simulink library "INP_IMU_ManOver"  (R2022a)
settings: Solver=VariableStepAuto  StartTime=0.0  StopTime=10.0  RelTol=1e-3
undefined symbols (not defined in the file): INP_IMU_p_ALatVehLoLim_mps2, INP_IMU_p_ALatVehMan_mps2, INP_IMU_p_ALatVehUpLim_mps2, INP_IMU_p_ALgtVehLoLim_mps2, INP_IMU_p_ALgtVehMan_mps2, INP_IMU_p_ALgtVehUpLim_mps2, INP_IMU_p_AVertVehLoLim_mps2, INP_IMU_p_AVertVehMan_mps2, INP_IMU_p_AVertVehUpLim_mps2, INP_IMU_p_SwtALatVehMan_na, INP_IMU_p_SwtALgtVehMan_na, INP_IMU_p_SwtAVertVehMan_na
libraries: simulink x3
settings Model: Creator=blatak  LastModifiedBy=blatak

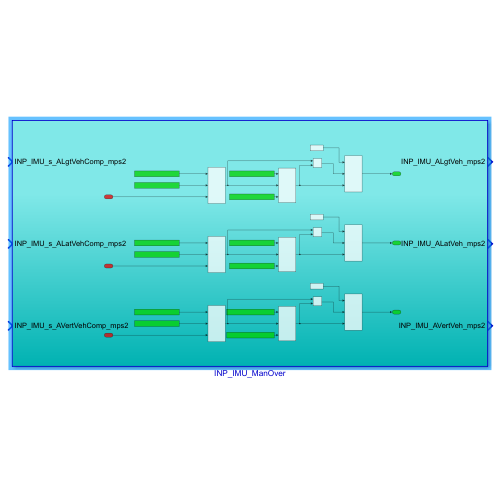
[thumbnail: Simulink's stored preview of the top-level diagram]
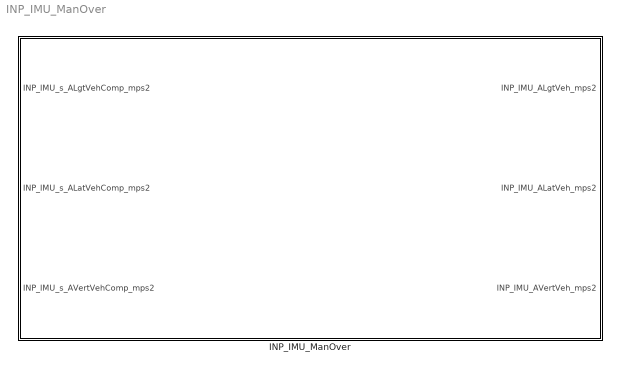
== system INP_IMU_ManOver ==
  INP_IMU_ManOver : Subsystem

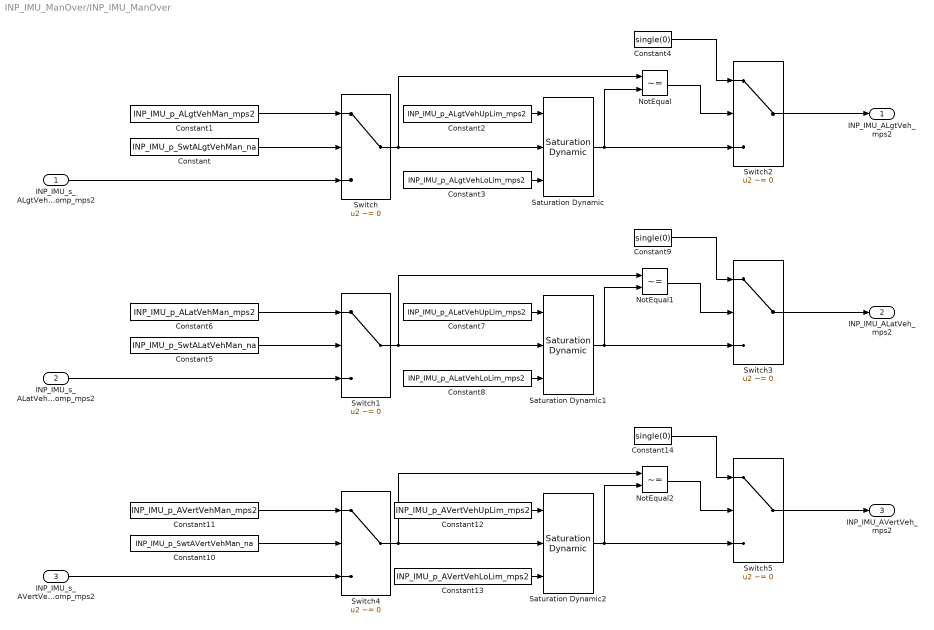
== system INP_IMU_ManOver/INP_IMU_ManOver ==
  INP_IMU_s_ALgtVehComp_mps2 : Inport
  INP_IMU_s_ALatVehComp_mps2 : Inport  Port=2
  INP_IMU_s_AVertVehComp_mps2 : Inport  Port=3
  Constant : Constant  Value=INP_IMU_p_SwtALgtVehMan_na
  Constant1 : Constant  Value=INP_IMU_p_ALgtVehMan_mps2
  Constant10 : Constant  Value=INP_IMU_p_SwtAVertVehMan_na
  Constant11 : Constant  Value=INP_IMU_p_AVertVehMan_mps2
  Constant12 : Constant  Value=INP_IMU_p_AVertVehUpLim_mps2
  Constant13 : Constant  Value=INP_IMU_p_AVertVehLoLim_mps2
  Constant14 : Constant  Value=single(0)
  Constant2 : Constant  Value=INP_IMU_p_ALgtVehUpLim_mps2
  Constant3 : Constant  Value=INP_IMU_p_ALgtVehLoLim_mps2
  Constant4 : Constant  Value=single(0)
  Constant5 : Constant  Value=INP_IMU_p_SwtALatVehMan_na
  Constant6 : Constant  Value=INP_IMU_p_ALatVehMan_mps2
  Constant7 : Constant  Value=INP_IMU_p_ALatVehUpLim_mps2
  Constant8 : Constant  Value=INP_IMU_p_ALatVehLoLim_mps2
  Constant9 : Constant  Value=single(0)
  NotEqual : RelationalOperator  Operator=~=  OutDataTypeStr=boolean  RndMeth=Simplest  InputSameDT=off
  NotEqual1 : RelationalOperator  Operator=~=  OutDataTypeStr=boolean  RndMeth=Simplest  InputSameDT=off
  NotEqual2 : RelationalOperator  Operator=~=  OutDataTypeStr=boolean  RndMeth=Simplest  InputSameDT=off
  Saturation Dynamic : simulink/Discontinuities/Saturation Dynamic  OutMin=[]  OutMax=[]  OutDataTypeStr=Inherit: Same as second input  OutDataType=fixdt(1, 16)  OutScaling=2^-10  DoSatur=off
  Saturation Dynamic1 : simulink/Discontinuities/Saturation Dynamic  OutMin=[]  OutMax=[]  OutDataTypeStr=Inherit: Same as second input  OutDataType=fixdt(1, 16)  OutScaling=2^-10  DoSatur=off
  Saturation Dynamic2 : simulink/Discontinuities/Saturation Dynamic  OutMin=[]  OutMax=[]  OutDataTypeStr=Inherit: Same as second input  OutDataType=fixdt(1, 16)  OutScaling=2^-10  DoSatur=off
  Switch{,1..5} (6 alike) : Switch  Criteria=u2 ~= 0  SaturateOnIntegerOverflow=off  InputSameDT=off
  INP_IMU_ALgtVeh_mps2 : Outport
  INP_IMU_ALatVeh_mps2 : Outport  Port=2
  INP_IMU_AVertVeh_mps2 : Outport  Port=3
  wires:
  Switch3/1 -> INP_IMU_ALatVeh_mps2/1
  Constant3/1 -> Saturation Dynamic/3
  Constant9/1 -> Switch3/1
  Saturation Dynamic1/1 -> Switch3/3, NotEqual1/2
  Constant4/1 -> Switch2/1
  Constant8/1 -> Saturation Dynamic1/3
  Switch1/1 -> NotEqual1/1, Saturation Dynamic1/2
  Constant7/1 -> Saturation Dynamic1/1
  NotEqual1/1 -> Switch3/2
  Constant2/1 -> Saturation Dynamic/1
  Constant/1 -> Switch/2
  Switch2/1 -> INP_IMU_ALgtVeh_mps2/1
  INP_IMU_s_ALgtVehComp_mps2/1 -> Switch/3
  Saturation Dynamic/1 -> Switch2/3, NotEqual/2
  INP_IMU_s_ALatVehComp_mps2/1 -> Switch1/3
  Constant6/1 -> Switch1/1
  Switch/1 -> NotEqual/1, Saturation Dynamic/2
  Constant5/1 -> Switch1/2
  NotEqual/1 -> Switch2/2
  Constant1/1 -> Switch/1
  Constant10/1 -> Switch4/2
  Constant12/1 -> Saturation Dynamic2/1
  Constant11/1 -> Switch4/1
  NotEqual2/1 -> Switch5/2
  INP_IMU_s_AVertVehComp_mps2/1 -> Switch4/3
  Saturation Dynamic2/1 -> Switch5/3, NotEqual2/2
  Switch5/1 -> INP_IMU_AVertVeh_mps2/1
  Constant14/1 -> Switch5/1
  Constant13/1 -> Saturation Dynamic2/3
  Switch4/1 -> NotEqual2/1, Saturation Dynamic2/2
